simulink model "openLoopBoiler_RF"  (R2017a)
settings: Solver=FixedStepAuto  StartTime=0.0  StopTime=simTime  FixedStep=Dt  RelTol=1e-3  EnableMultiTasking=on
values from neighbouring files (symbols this model uses):
  D0 = 35.783396242    [cic2017_fase1_boiler.mat]    (also in compare_rf_boiler.m = 35.7834; control_Caldera_3004.m = 35.7834; mpcGASimulink_2205_dummy.m = 35.7834; mpc_design_parameters_0206.mat = 35.7834)
  Dt = 1    [compare_rf_boiler.m]    (also in control_Caldera_3004.m = 0.5; mpcBoiler_0206.m; mpcBoiler_2805.m; mpcBoiler_closed_loop_0206.m)
  effectiveReactionTime = 5    [delayParameters_0405.mat]
  make = makeMatrix(m,:)    [compare_rf_boiler.m]    (also in mpcGASimulink_2205_dummy.m = [1 0 1 1]; rf_boiler_simulateScript.m; simScript.m = [1 0 1 1]; testBigData.m)
  numCV = length(Y0)    [compare_rf_boiler.m]    (also in mpcGASimulink_2205_dummy.m; mpc_design_parameters_0206.mat = 3; mpc_design_parameters_0606.mat = 3; mpc_design_parameters_0706.mat = 3)
  numDV = length(D0)    [compare_rf_boiler.m]    (also in delayParameters_0405.mat = 1; delayParameters_0706.mat = 1; delayParameters_2805.mat = 1; mpcGASimulink_2205_dummy.m)
  numMV = length(U0)    [compare_rf_boiler.m]    (also in delayParameters_0405.mat = 3; delayParameters_0706.mat = 3; delayParameters_2805.mat = 3; mpcGASimulink_2205_dummy.m)
  U0 = [32.9815865199 46.2282063472 25.3416381967]    [cic2017_fase1_boiler.mat]    (also in compare_rf_boiler.m = [32.9816   46.2282   25.3416]; control_Caldera_3004.m = [32.9816   46.2282   25.3416]; mpcGASimulink_2205_dummy.m = [32.9816   46.2282   25.3416]; mpc_design_parameters_0206.mat = [32.9816 46.2282 25.3416])
  uRecSize = max(max(delayUMatrix))    [mpcGASimulink_2205_dummy.m]    (also in trialsRF_Simulink.m)
  Y0 = [41.4119839556 28.7552838432 38.6036799989]    [cic2017_fase1_boiler.mat]    (also in compare_rf_boiler.m = [41.4120   28.7553   38.6037]; control_Caldera_3004.m = [41.4120   28.7553   38.6037]; mpcGASimulink_2205_dummy.m = [41.4120   28.7553   38.6037]; mpc_design_parameters_0206.mat = [41.412 28.7553 38.6037])
  yRecSize = max(max(delayYMatrix))    [mpcGASimulink_2205_dummy.m]    (also in trialsRF_Simulink.m)
undefined symbols (not defined in the file or in its folder): delayUMatrix, delayYMatrix
settings Model: Creator=Pablo Diaz  LastModifiedBy=Felipe
settings OptimizationCC: LifeSpan=inf
settings DebuggingCC: SFUnexpectedBacktrackingDiag=warning  SFNoUnconditionalDefaultTransitionDiag=warning  SFExecutionAtInitializationDiag=none
settings GRTTargetCC: TargetLangStandard=C89/C90 (ANSI)
settings ConfigComp: CovMetricSettings=dw  CovHtmlReporting=on  CovSaveCumulativeToWorkspaceVar=on  CovSaveSingleToWorkspaceVar=on  CovExternalEMLEnable=off

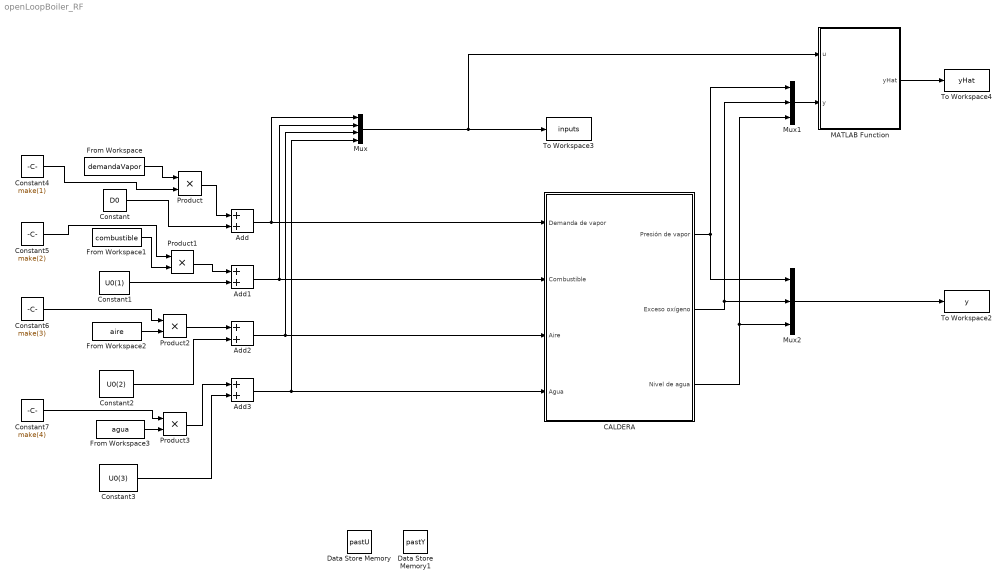
== system openLoopBoiler_RF ==
  Add{,1..3} (4 alike) : Sum
  CALDERA : Subsystem
  Constant : Constant  Value=D0
  Constant1 : Constant  Value=U0(1)
  Constant2 : Constant  Value=U0(2)
  Constant3 : Constant  Value=U0(3)
  Constant4 : Constant  Value=make(1)
  Constant5 : Constant  Value=make(2)
  Constant6 : Constant  Value=make(3)
  Constant7 : Constant  Value=make(4)
  Data Store Memory : DataStoreMemory  DataStoreName=pastU  ReadBeforeWriteMsg=warning  WriteAfterWriteMsg=warning  WriteAfterReadMsg=warning  InitialValue=[D0 U0]'*ones(1,uRecSize*effectiveReactionTime);  VectorParams1D=off  ShowAdditionalParam=off  OutDataTypeStr=double
  Data Store Memory1 : DataStoreMemory  DataStoreName=pastY  ReadBeforeWriteMsg=warning  WriteAfterWriteMsg=warning  WriteAfterReadMsg=warning  InitialValue=Y0'*ones(1,yRecSize*effectiveReactionTime)  VectorParams1D=off  ShowAdditionalParam=off  OutDataTypeStr=double
  From Workspace : FromWorkspace  VariableName=demandaVapor  SampleTime=Dt
  From Workspace1 : FromWorkspace  VariableName=combustible  SampleTime=Dt
  From Workspace2 : FromWorkspace  VariableName=aire  SampleTime=Dt
  From Workspace3 : FromWorkspace  VariableName=agua  SampleTime=Dt
  MATLAB Function : MATLAB Function  TreatAsAtomicUnit=on
  Mux : Mux
  Mux1 : Mux  Inputs=3
  Mux2 : Mux  Inputs=3
  Product{,1..3} (4 alike) : Product
  To Workspace2 : ToWorkspace  VariableName=y  SaveFormat=Structure With Time  SampleTime=-1
  To Workspace3 : ToWorkspace  VariableName=inputs  SaveFormat=Structure With Time  SampleTime=-1
  To Workspace4 : ToWorkspace  VariableName=yHat  SaveFormat=Structure With Time  SampleTime=-1
  wires:
  CALDERA/2(Exceso oxígeno) -> Mux2/2, Mux1/2
  From Workspace/1 -> Product/1
  Constant/1 -> Add/2
  From Workspace1/1 -> Product1/2
  Constant1/1 -> Add1/2
  From Workspace2/1 -> Product2/2
  Add2/1 -> Mux/3, CALDERA/3(Aire)
  Constant2/1 -> Add2/2
  From Workspace3/1 -> Product3/2
  Add3/1 -> Mux/4, CALDERA/4(Agua)
  Constant3/1 -> Add3/2
  Constant4/1 -> Product/2
  Product/1 -> Add/1
  Constant5/1 -> Product1/1
  Product1/1 -> Add1/1
  Constant6/1 -> Product2/1
  Product2/1 -> Add2/1
  Product3/1 -> Add3/1
  Constant7/1 -> Product3/1
  Add1/1 -> Mux/2, CALDERA/2(Combustible)
  Add/1 -> Mux/1, CALDERA/1(Demanda de vapor)
  Mux/1 -> MATLAB Function/1(u), To Workspace3/1
  CALDERA/1(Presión de vapor) -> Mux2/1, Mux1/1
  MATLAB Function/1(yHat) -> To Workspace4/1
  CALDERA/3(Nivel de agua) -> Mux1/3, Mux2/3
  Mux1/1 -> MATLAB Function/2(y)
  Mux2/1 -> To Workspace2/1

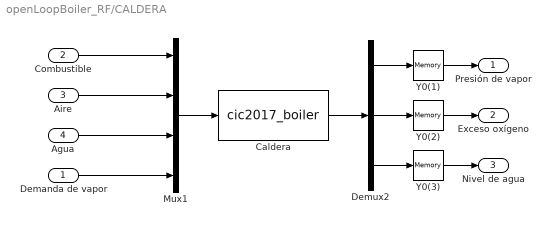
== system openLoopBoiler_RF/CALDERA ==
  Demanda de vapor : Inport
  Combustible : Inport  Port=2
  Aire : Inport  Port=3
  Agua : Inport  Port=4
  Caldera : S-Function  FunctionName=cic2017_boiler  Parameters=Y0,[U0 D0]  SFunctionDeploymentMode=off  EnableBusSupport=off
  Demux2 : Demux  Outputs=3
  Mux1 : Mux
  Y0(1) : Memory  X0=Y0(1)
  Y0(2) : Memory  X0=Y0(2)
  Y0(3) : Memory  X0=Y0(3)
  Presión de vapor : Outport
  Exceso oxígeno : Outport  Port=2
  Nivel de agua : Outport  Port=3
  wires:
  Caldera/1 -> Demux2/1
  Aire/1 -> Mux1/2
  Agua/1 -> Mux1/3
  Demanda de vapor/1 -> Mux1/4
  Combustible/1 -> Mux1/1
  Mux1/1 -> Caldera/1
  Demux2/1 -> Y0(1)/1
  Demux2/2 -> Y0(2)/1
  Demux2/3 -> Y0(3)/1
  Y0(1)/1 -> Presión de vapor/1
  Y0(2)/1 -> Exceso oxígeno/1
  Y0(3)/1 -> Nivel de agua/1

== matlab function openLoopBoiler_RF/MATLAB Function ==
  data: u input; y input; yHat output size=[3 1]; pastU data_store_memory; pastY data_store_memory; effectiveReactionTime parameter; delayUMatrix parameter; numMV parameter; numDV parameter; numCV parameter; delayYMatrix parameter
function yHat = predictorSimulink(u,y,effectiveReactionTime, delayUMatrix, numMV, numDV, numCV, delayYMatrix)

coder.extrinsic('predictRF_Y1_mex');
coder.extrinsic('predictRF_Y2_mex');
coder.extrinsic('predictRF_Y3_mex');
global pastU
global pastY
% u: vector containing [dv mv(1) mv(2) mv(3)];0
% y: vector containing [y(1) y(2) y(3)]
yHat = zeros(numCV,1);
pastY(:,2:end) = pastY(:,1:end-1);
pastY(:,1) = y;
for i = 1:numCV
    % Chooses best-model specific delay in Y for output i
    delayY = delayYMatrix(i,i);
%     X = [y(i) pastY(i,[1:delayY]*effectiveReactionTime)];
    X = [pastY(i,[1:delayY]*effectiveReactionTime)];
    % Chooses best-model specific delay in DV for output i
    for j = 1:numDV
        delayU = delayUMatrix(i,j);
        X = [X u(j) pastU(j,[1:delayU]*effectiveReactionTime)];
    end
    % Chooses best-model specific delay in MV for output i
    for j = 1+numDV:numMV+numDV
        delayU = delayUMatrix(i,j);
        X = [X u(j) pastU(j,[1:delayU]*effectiveReactionTime)];
    end
    % Predict
    switch i
        case 1
            yHat(i) = predictRF_Y1_mex(X,100,10);
        case 2
            yHat(i) = predictRF_Y2_mex(X,100,10);
        case 3
            yHat(i) = predictRF_Y3_mex(X,100,10);
    end
end
pastU(:,2:end) = pastU(:,1:end-1);
pastU(:,1) = u;
